simulink model "ROSCO"  (R2023a)
settings: Solver=ode4  StartTime=0.0  StopTime=TMax  FixedStep=simu.dt  RelTol=1e-3  EnableMultiTasking=on
undefined symbols (not defined in the file): DiscIntNeverNeededParam, F, OutList, Parameter, R, rpm2radps, simu, strmatch
libraries: simulink x10
(part 2 of 3)

== system ROSCO/Cyclic Pitch controller/1P Cyclic Pitch Controller1/1P IPCDQ Filtering1/Moving 3P Notch Man Z ==
  Input : Inport
  GenSpeedIN : Inport  Port=2
  Gain : Gain  Gain=1/Parameter.Turbine.G * rpm2radps(1) * 3
  Moving 3P Filt Manual : Subsystem
  Slow Low Pass for Param : DiscreteStateSpace  A=Parameter.Control.cIPC.dLPF_slow.a  B=Parameter.Control.cIPC.dLPF_slow.b  C=Parameter.Control.cIPC.dLPF_slow.c  D=Parameter.Control.cIPC.dLPF_slow.d  SampleTime=Parameter.Control.DT
  Output : Outport  VectorParamsAs1DForOutWhenUnconnected=off
  wires:
  Moving 3P Filt Manual/1(Out1) -> Output/1
  GenSpeedIN/1 -> Slow Low Pass for Param/1
  Input/1 -> Moving 3P Filt Manual/1(u)
  Gain/1 -> Moving 3P Filt Manual/2(rot speed (rad/s))
  Slow Low Pass for Param/1 -> Gain/1

== system ROSCO/Cyclic Pitch controller/1P Cyclic Pitch Controller1/1P IPCDQ Filtering1/Moving 6P Notch Man Y ==
  Input : Inport
  GenSpeedIN : Inport  Port=2
  Gain : Gain  Gain=1/Parameter.Turbine.G * rpm2radps(1) * 3
  Moving 6P Filt Manual : Subsystem
  Slow Low Pass for Param : DiscreteStateSpace  A=Parameter.Control.cIPC.dLPF_slow.a  B=Parameter.Control.cIPC.dLPF_slow.b  C=Parameter.Control.cIPC.dLPF_slow.c  D=Parameter.Control.cIPC.dLPF_slow.d  SampleTime=Parameter.Control.DT
  Output : Outport  VectorParamsAs1DForOutWhenUnconnected=off
  wires:
  Moving 6P Filt Manual/1(Out1) -> Output/1
  GenSpeedIN/1 -> Slow Low Pass for Param/1
  Input/1 -> Moving 6P Filt Manual/1(u)
  Gain/1 -> Moving 6P Filt Manual/2(rot speed (rad/s))
  Slow Low Pass for Param/1 -> Gain/1

== system ROSCO/Cyclic Pitch controller/1P Cyclic Pitch Controller1/1P IPCDQ Filtering1/Moving 6P Notch Man Z ==
  Input : Inport
  GenSpeedIN : Inport  Port=2
  Gain : Gain  Gain=1/Parameter.Turbine.G * rpm2radps(1) * 3
  Moving 6P Filt Manual : Subsystem
  Slow Low Pass for Param : DiscreteStateSpace  A=Parameter.Control.cIPC.dLPF_slow.a  B=Parameter.Control.cIPC.dLPF_slow.b  C=Parameter.Control.cIPC.dLPF_slow.c  D=Parameter.Control.cIPC.dLPF_slow.d  SampleTime=Parameter.Control.DT
  Output : Outport  VectorParamsAs1DForOutWhenUnconnected=off
  wires:
  Slow Low Pass for Param/1 -> Gain/1
  Gain/1 -> Moving 6P Filt Manual/2(rot speed (rad/s))
  Input/1 -> Moving 6P Filt Manual/1(u)
  GenSpeedIN/1 -> Slow Low Pass for Param/1
  Moving 6P Filt Manual/1(Out1) -> Output/1

== system ROSCO/Cyclic Pitch controller/1P Cyclic Pitch Controller1/M0 Signal Proc.1/Moving 1P Notch Man ==
  Input : Inport
  GenSpeedIN : Inport  Port=2
  Gain : Gain  Gain=1/Parameter.Turbine.G * rpm2radps(1)
  Moving 1P Filt Manual : Subsystem
  Slow Low Pass for Param : DiscreteStateSpace  A=Parameter.Control.cIPC.dLPF_slow.a  B=Parameter.Control.cIPC.dLPF_slow.b  C=Parameter.Control.cIPC.dLPF_slow.c  D=Parameter.Control.cIPC.dLPF_slow.d  SampleTime=Parameter.Control.DT
  Output : Outport  VectorParamsAs1DForOutWhenUnconnected=off
  wires:
  GenSpeedIN/1 -> Slow Low Pass for Param/1
  Input/1 -> Moving 1P Filt Manual/1(u)
  Gain/1 -> Moving 1P Filt Manual/2(rot speed (rad/s))
  Slow Low Pass for Param/1 -> Gain/1
  Moving 1P Filt Manual/1(Out1) -> Output/1

== system ROSCO/Cyclic Pitch controller/1P Cyclic Pitch Controller1/M0 Signal Proc.1/Moving 3P Notch Man ==
  Input : Inport
  GenSpeedIN : Inport  Port=2
  Gain : Gain  Gain=1/Parameter.Turbine.G * rpm2radps(1) * 3
  Moving 3P Filt Manual : Subsystem
  Slow Low Pass for Param : DiscreteStateSpace  A=Parameter.Control.cIPC.dLPF_slow.a  B=Parameter.Control.cIPC.dLPF_slow.b  C=Parameter.Control.cIPC.dLPF_slow.c  D=Parameter.Control.cIPC.dLPF_slow.d  SampleTime=Parameter.Control.DT
  Output : Outport  VectorParamsAs1DForOutWhenUnconnected=off
  wires:
  Slow Low Pass for Param/1 -> Gain/1
  Gain/1 -> Moving 3P Filt Manual/2(rot speed (rad/s))
  Input/1 -> Moving 3P Filt Manual/1(u)
  GenSpeedIN/1 -> Slow Low Pass for Param/1
  Moving 3P Filt Manual/1(Out1) -> Output/1

== system ROSCO/Cyclic Pitch controller/2P Cyclic Pitch Controller2/1P IPCDQ Filtering1/Moving 3P Notch Man Y ==
  Input : Inport
  GenSpeedIN : Inport  Port=2
  Gain : Gain  Gain=1/Parameter.Turbine.G * rpm2radps(1) * 3
  Moving 3P Filt Manual : Subsystem
  Slow Low Pass for Param : DiscreteStateSpace  A=Parameter.Control.cIPC.dLPF_slow.a  B=Parameter.Control.cIPC.dLPF_slow.b  C=Parameter.Control.cIPC.dLPF_slow.c  D=Parameter.Control.cIPC.dLPF_slow.d  SampleTime=Parameter.Control.DT
  Output : Outport  VectorParamsAs1DForOutWhenUnconnected=off
  wires:
  Slow Low Pass for Param/1 -> Gain/1
  Gain/1 -> Moving 3P Filt Manual/2(rot speed (rad/s))
  Input/1 -> Moving 3P Filt Manual/1(u)
  GenSpeedIN/1 -> Slow Low Pass for Param/1
  Moving 3P Filt Manual/1(Out1) -> Output/1

== system ROSCO/Cyclic Pitch controller/2P Cyclic Pitch Controller2/1P IPCDQ Filtering1/Moving 3P Notch Man Z ==
  Input : Inport
  GenSpeedIN : Inport  Port=2
  Gain : Gain  Gain=1/Parameter.Turbine.G * rpm2radps(1) * 3
  Moving 3P Filt Manual : Subsystem
  Slow Low Pass for Param : DiscreteStateSpace  A=Parameter.Control.cIPC.dLPF_slow.a  B=Parameter.Control.cIPC.dLPF_slow.b  C=Parameter.Control.cIPC.dLPF_slow.c  D=Parameter.Control.cIPC.dLPF_slow.d  SampleTime=Parameter.Control.DT
  Output : Outport  VectorParamsAs1DForOutWhenUnconnected=off
  wires:
  Moving 3P Filt Manual/1(Out1) -> Output/1
  GenSpeedIN/1 -> Slow Low Pass for Param/1
  Input/1 -> Moving 3P Filt Manual/1(u)
  Gain/1 -> Moving 3P Filt Manual/2(rot speed (rad/s))
  Slow Low Pass for Param/1 -> Gain/1

== system ROSCO/Cyclic Pitch controller/2P Cyclic Pitch Controller2/1P IPCDQ Filtering1/Moving 6P Notch Man Y ==
  Input : Inport
  GenSpeedIN : Inport  Port=2
  Gain : Gain  Gain=1/Parameter.Turbine.G * rpm2radps(1) * 3
  Moving 6P Filt Manual : Subsystem
  Slow Low Pass for Param : DiscreteStateSpace  A=Parameter.Control.cIPC.dLPF_slow.a  B=Parameter.Control.cIPC.dLPF_slow.b  C=Parameter.Control.cIPC.dLPF_slow.c  D=Parameter.Control.cIPC.dLPF_slow.d  SampleTime=Parameter.Control.DT
  Output : Outport  VectorParamsAs1DForOutWhenUnconnected=off
  wires:
  Moving 6P Filt Manual/1(Out1) -> Output/1
  GenSpeedIN/1 -> Slow Low Pass for Param/1
  Input/1 -> Moving 6P Filt Manual/1(u)
  Gain/1 -> Moving 6P Filt Manual/2(rot speed (rad/s))
  Slow Low Pass for Param/1 -> Gain/1

== system ROSCO/Cyclic Pitch controller/2P Cyclic Pitch Controller2/1P IPCDQ Filtering1/Moving 6P Notch Man Z ==
  Input : Inport
  GenSpeedIN : Inport  Port=2
  Gain : Gain  Gain=1/Parameter.Turbine.G * rpm2radps(1) * 3
  Moving 6P Filt Manual : Subsystem
  Slow Low Pass for Param : DiscreteStateSpace  A=Parameter.Control.cIPC.dLPF_slow.a  B=Parameter.Control.cIPC.dLPF_slow.b  C=Parameter.Control.cIPC.dLPF_slow.c  D=Parameter.Control.cIPC.dLPF_slow.d  SampleTime=Parameter.Control.DT
  Output : Outport  VectorParamsAs1DForOutWhenUnconnected=off
  wires:
  Slow Low Pass for Param/1 -> Gain/1
  Gain/1 -> Moving 6P Filt Manual/2(rot speed (rad/s))
  Input/1 -> Moving 6P Filt Manual/1(u)
  GenSpeedIN/1 -> Slow Low Pass for Param/1
  Moving 6P Filt Manual/1(Out1) -> Output/1

== system ROSCO/Cyclic Pitch controller/2P Cyclic Pitch Controller2/M0 Signal Proc.1/Moving 1P Notch Man ==
  Input : Inport
  GenSpeedIN : Inport  Port=2
  Gain : Gain  Gain=1/Parameter.Turbine.G * rpm2radps(1)
  Moving 1P Filt Manual : Subsystem
  Slow Low Pass for Param : DiscreteStateSpace  A=Parameter.Control.cIPC.dLPF_slow.a  B=Parameter.Control.cIPC.dLPF_slow.b  C=Parameter.Control.cIPC.dLPF_slow.c  D=Parameter.Control.cIPC.dLPF_slow.d  SampleTime=Parameter.Control.DT
  Output : Outport  VectorParamsAs1DForOutWhenUnconnected=off
  wires:
  GenSpeedIN/1 -> Slow Low Pass for Param/1
  Input/1 -> Moving 1P Filt Manual/1(u)
  Gain/1 -> Moving 1P Filt Manual/2(rot speed (rad/s))
  Slow Low Pass for Param/1 -> Gain/1
  Moving 1P Filt Manual/1(Out1) -> Output/1

== system ROSCO/Cyclic Pitch controller/2P Cyclic Pitch Controller2/M0 Signal Proc.1/Moving 3P Notch Man ==
  Input : Inport
  GenSpeedIN : Inport  Port=2
  Gain : Gain  Gain=1/Parameter.Turbine.G * rpm2radps(1) * 3
  Moving 3P Filt Manual : Subsystem
  Slow Low Pass for Param : DiscreteStateSpace  A=Parameter.Control.cIPC.dLPF_slow.a  B=Parameter.Control.cIPC.dLPF_slow.b  C=Parameter.Control.cIPC.dLPF_slow.c  D=Parameter.Control.cIPC.dLPF_slow.d  SampleTime=Parameter.Control.DT
  Output : Outport  VectorParamsAs1DForOutWhenUnconnected=off
  wires:
  Slow Low Pass for Param/1 -> Gain/1
  Gain/1 -> Moving 3P Filt Manual/2(rot speed (rad/s))
  Input/1 -> Moving 3P Filt Manual/1(u)
  GenSpeedIN/1 -> Slow Low Pass for Param/1
  Moving 3P Filt Manual/1(Out1) -> Output/1

== system ROSCO/Cyclic Pitch controller/1P Cyclic Pitch Controller1/1P IPCDQ Filtering1/Moving 3P Notch Man Y/Moving 3P Filt Manual ==
  u : Inport
  rot speed (rad/s) : Inport  Port=2
  Den LPV : Subsystem
  Discrete Filter : DiscreteFilter  NumeratorSource=Input port  DenominatorSource=Input port  a0EqualsOne=on
      settings: InputPortMap=u0,p1,p3
  Num LPV : Subsystem
  Out1 : Outport  VectorParamsAs1DForOutWhenUnconnected=off
  wires:
  u/1 -> Discrete Filter/1
  Num LPV/1(b) -> Discrete Filter/2
  Discrete Filter/1 -> Out1/1
  rot speed (rad/s)/1 -> Den LPV/1(rot speed (rad/s)), Num LPV/1(rot speed (rad/s))
  Den LPV/1(a) -> Discrete Filter/3

== system ROSCO/Cyclic Pitch controller/1P Cyclic Pitch Controller1/1P IPCDQ Filtering1/Moving 3P Notch Man Z/Moving 3P Filt Manual ==
  u : Inport
  rot speed (rad/s) : Inport  Port=2
  Den LPV : Subsystem
  Discrete Filter : DiscreteFilter  NumeratorSource=Input port  DenominatorSource=Input port  a0EqualsOne=on
      settings: InputPortMap=u0,p1,p3
  Num LPV : Subsystem
  Out1 : Outport  VectorParamsAs1DForOutWhenUnconnected=off
  wires:
  Den LPV/1(a) -> Discrete Filter/3
  rot speed (rad/s)/1 -> Num LPV/1(rot speed (rad/s)), Den LPV/1(rot speed (rad/s))
  Discrete Filter/1 -> Out1/1
  Num LPV/1(b) -> Discrete Filter/2
  u/1 -> Discrete Filter/1

== system ROSCO/Cyclic Pitch controller/1P Cyclic Pitch Controller1/1P IPCDQ Filtering1/Moving 6P Notch Man Y/Moving 6P Filt Manual ==
  u : Inport
  rot speed (rad/s) : Inport  Port=2
  Den LPV : Subsystem
  Discrete Filter : DiscreteFilter  NumeratorSource=Input port  DenominatorSource=Input port  a0EqualsOne=on
      settings: InputPortMap=u0,p1,p3
  Num LPV : Subsystem
  Out1 : Outport  VectorParamsAs1DForOutWhenUnconnected=off
  wires:
  Den LPV/1(a) -> Discrete Filter/3
  rot speed (rad/s)/1 -> Num LPV/1(rot speed (rad/s)), Den LPV/1(rot speed (rad/s))
  Discrete Filter/1 -> Out1/1
  Num LPV/1(b) -> Discrete Filter/2
  u/1 -> Discrete Filter/1

== system ROSCO/Cyclic Pitch controller/1P Cyclic Pitch Controller1/1P IPCDQ Filtering1/Moving 6P Notch Man Z/Moving 6P Filt Manual ==
  u : Inport
  rot speed (rad/s) : Inport  Port=2
  Den LPV : Subsystem
  Discrete Filter : DiscreteFilter  NumeratorSource=Input port  DenominatorSource=Input port  a0EqualsOne=on
      settings: InputPortMap=u0,p1,p3
  Num LPV : Subsystem
  Out1 : Outport  VectorParamsAs1DForOutWhenUnconnected=off
  wires:
  u/1 -> Discrete Filter/1
  Num LPV/1(b) -> Discrete Filter/2
  Discrete Filter/1 -> Out1/1
  rot speed (rad/s)/1 -> Den LPV/1(rot speed (rad/s)), Num LPV/1(rot speed (rad/s))
  Den LPV/1(a) -> Discrete Filter/3

== system ROSCO/Cyclic Pitch controller/1P Cyclic Pitch Controller1/M0 Signal Proc.1/Moving 1P Notch Man/Moving 1P Filt Manual ==
  u : Inport
  rot speed (rad/s) : Inport  Port=2
  Den LPV : Subsystem
  Discrete Filter : DiscreteFilter  NumeratorSource=Input port  DenominatorSource=Input port  a0EqualsOne=on
      settings: InputPortMap=u0,p1,p3
  Num LPV : Subsystem
  Out1 : Outport  VectorParamsAs1DForOutWhenUnconnected=off
  wires:
  Den LPV/1(a) -> Discrete Filter/3
  rot speed (rad/s)/1 -> Num LPV/1(rot speed (rad/s)), Den LPV/1(rot speed (rad/s))
  Discrete Filter/1 -> Out1/1
  Num LPV/1(b) -> Discrete Filter/2
  u/1 -> Discrete Filter/1

== system ROSCO/Cyclic Pitch controller/1P Cyclic Pitch Controller1/M0 Signal Proc.1/Moving 3P Notch Man/Moving 3P Filt Manual ==
  u : Inport
  rot speed (rad/s) : Inport  Port=2
  Den LPV : Subsystem
  Discrete Filter : DiscreteFilter  NumeratorSource=Input port  DenominatorSource=Input port  a0EqualsOne=on
      settings: InputPortMap=u0,p1,p3
  Num LPV : Subsystem
  Out1 : Outport  VectorParamsAs1DForOutWhenUnconnected=off
  wires:
  u/1 -> Discrete Filter/1
  Num LPV/1(b) -> Discrete Filter/2
  Discrete Filter/1 -> Out1/1
  rot speed (rad/s)/1 -> Den LPV/1(rot speed (rad/s)), Num LPV/1(rot speed (rad/s))
  Den LPV/1(a) -> Discrete Filter/3

== system ROSCO/Cyclic Pitch controller/2P Cyclic Pitch Controller2/1P IPCDQ Filtering1/Moving 3P Notch Man Y/Moving 3P Filt Manual ==
  u : Inport
  rot speed (rad/s) : Inport  Port=2
  Den LPV : Subsystem
  Discrete Filter : DiscreteFilter  NumeratorSource=Input port  DenominatorSource=Input port  a0EqualsOne=on
      settings: InputPortMap=u0,p1,p3
  Num LPV : Subsystem
  Out1 : Outport  VectorParamsAs1DForOutWhenUnconnected=off
  wires:
  u/1 -> Discrete Filter/1
  Num LPV/1(b) -> Discrete Filter/2
  Discrete Filter/1 -> Out1/1
  rot speed (rad/s)/1 -> Den LPV/1(rot speed (rad/s)), Num LPV/1(rot speed (rad/s))
  Den LPV/1(a) -> Discrete Filter/3

== system ROSCO/Cyclic Pitch controller/2P Cyclic Pitch Controller2/1P IPCDQ Filtering1/Moving 3P Notch Man Z/Moving 3P Filt Manual ==
  u : Inport
  rot speed (rad/s) : Inport  Port=2
  Den LPV : Subsystem
  Discrete Filter : DiscreteFilter  NumeratorSource=Input port  DenominatorSource=Input port  a0EqualsOne=on
      settings: InputPortMap=u0,p1,p3
  Num LPV : Subsystem
  Out1 : Outport  VectorParamsAs1DForOutWhenUnconnected=off
  wires:
  Den LPV/1(a) -> Discrete Filter/3
  rot speed (rad/s)/1 -> Num LPV/1(rot speed (rad/s)), Den LPV/1(rot speed (rad/s))
  Discrete Filter/1 -> Out1/1
  Num LPV/1(b) -> Discrete Filter/2
  u/1 -> Discrete Filter/1

== system ROSCO/Cyclic Pitch controller/2P Cyclic Pitch Controller2/1P IPCDQ Filtering1/Moving 6P Notch Man Y/Moving 6P Filt Manual ==
  u : Inport
  rot speed (rad/s) : Inport  Port=2
  Den LPV : Subsystem
  Discrete Filter : DiscreteFilter  NumeratorSource=Input port  DenominatorSource=Input port  a0EqualsOne=on
      settings: InputPortMap=u0,p1,p3
  Num LPV : Subsystem
  Out1 : Outport  VectorParamsAs1DForOutWhenUnconnected=off
  wires:
  Den LPV/1(a) -> Discrete Filter/3
  rot speed (rad/s)/1 -> Num LPV/1(rot speed (rad/s)), Den LPV/1(rot speed (rad/s))
  Discrete Filter/1 -> Out1/1
  Num LPV/1(b) -> Discrete Filter/2
  u/1 -> Discrete Filter/1

== system ROSCO/Cyclic Pitch controller/2P Cyclic Pitch Controller2/1P IPCDQ Filtering1/Moving 6P Notch Man Z/Moving 6P Filt Manual ==
  u : Inport
  rot speed (rad/s) : Inport  Port=2
  Den LPV : Subsystem
  Discrete Filter : DiscreteFilter  NumeratorSource=Input port  DenominatorSource=Input port  a0EqualsOne=on
      settings: InputPortMap=u0,p1,p3
  Num LPV : Subsystem
  Out1 : Outport  VectorParamsAs1DForOutWhenUnconnected=off
  wires:
  u/1 -> Discrete Filter/1
  Num LPV/1(b) -> Discrete Filter/2
  Discrete Filter/1 -> Out1/1
  rot speed (rad/s)/1 -> Den LPV/1(rot speed (rad/s)), Num LPV/1(rot speed (rad/s))
  Den LPV/1(a) -> Discrete Filter/3

== system ROSCO/Cyclic Pitch controller/2P Cyclic Pitch Controller2/M0 Signal Proc.1/Moving 1P Notch Man/Moving 1P Filt Manual ==
  u : Inport
  rot speed (rad/s) : Inport  Port=2
  Den LPV : Subsystem
  Discrete Filter : DiscreteFilter  NumeratorSource=Input port  DenominatorSource=Input port  a0EqualsOne=on
      settings: InputPortMap=u0,p1,p3
  Num LPV : Subsystem
  Out1 : Outport  VectorParamsAs1DForOutWhenUnconnected=off
  wires:
  Den LPV/1(a) -> Discrete Filter/3
  rot speed (rad/s)/1 -> Num LPV/1(rot speed (rad/s)), Den LPV/1(rot speed (rad/s))
  Discrete Filter/1 -> Out1/1
  Num LPV/1(b) -> Discrete Filter/2
  u/1 -> Discrete Filter/1

== system ROSCO/Cyclic Pitch controller/2P Cyclic Pitch Controller2/M0 Signal Proc.1/Moving 3P Notch Man/Moving 3P Filt Manual ==
  u : Inport
  rot speed (rad/s) : Inport  Port=2
  Den LPV : Subsystem
  Discrete Filter : DiscreteFilter  NumeratorSource=Input port  DenominatorSource=Input port  a0EqualsOne=on
      settings: InputPortMap=u0,p1,p3
  Num LPV : Subsystem
  Out1 : Outport  VectorParamsAs1DForOutWhenUnconnected=off
  wires:
  u/1 -> Discrete Filter/1
  Num LPV/1(b) -> Discrete Filter/2
  Discrete Filter/1 -> Out1/1
  rot speed (rad/s)/1 -> Den LPV/1(rot speed (rad/s)), Num LPV/1(rot speed (rad/s))
  Den LPV/1(a) -> Discrete Filter/3

== system ROSCO/Cyclic Pitch controller/1P Cyclic Pitch Controller1/1P IPCDQ Filtering1/Moving 3P Notch Man Y/Moving 3P Filt Manual/Den LPV ==
  rot speed (rad/s) : Inport
  1-D Lookup Table : Lookup_n-D  NumberOfTableDimensions=1  BreakpointsForDimension1=Parameter.Control.cIPC.PSM0_NF_3P.om_3P  BeginIndexSearchUsingPreviousIndexResult=on  Table=Parameter.Control.cIPC.PSM0_NF_3P.a_2  ExtrapMethod=Clip  InternalRulePriority=Speed  RndMeth=Simplest
  1-D Lookup Table1 : Lookup_n-D  NumberOfTableDimensions=1  BreakpointsForDimension1=Parameter.Control.cIPC.PSM0_NF_3P.om_3P  BeginIndexSearchUsingPreviousIndexResult=on  Table=Parameter.Control.cIPC.PSM0_NF_3P.a_1  ExtrapMethod=Clip  InternalRulePriority=Speed  RndMeth=Simplest
  1-D Lookup Table2 : Lookup_n-D  NumberOfTableDimensions=1  BreakpointsForDimension1=Parameter.Control.cIPC.PSM0_NF_3P.om_3P  BeginIndexSearchUsingPreviousIndexResult=on  Table=Parameter.Control.cIPC.PSM0_NF_3P.a_0  ExtrapMethod=Clip  InternalRulePriority=Speed  RndMeth=Simplest
  Mux : Mux  Inputs=3
  a : Outport  VectorParamsAs1DForOutWhenUnconnected=off
  wires:
  1-D Lookup Table/1 -> Mux/1
  1-D Lookup Table1/1 -> Mux/2
  Mux/1 -> a/1
  rot speed (rad/s)/1 -> 1-D Lookup Table2/1, 1-D Lookup Table/1, 1-D Lookup Table1/1
  1-D Lookup Table2/1 -> Mux/3

== system ROSCO/Cyclic Pitch controller/1P Cyclic Pitch Controller1/1P IPCDQ Filtering1/Moving 3P Notch Man Y/Moving 3P Filt Manual/Num LPV ==
  rot speed (rad/s) : Inport
  1-D Lookup Table : Lookup_n-D  NumberOfTableDimensions=1  BreakpointsForDimension1=Parameter.Control.cIPC.PSM0_NF_3P.om_3P  BeginIndexSearchUsingPreviousIndexResult=on  Table=Parameter.Control.cIPC.PSM0_NF_3P.b_2  ExtrapMethod=Clip  InternalRulePriority=Speed  RndMeth=Simplest
  1-D Lookup Table1 : Lookup_n-D  NumberOfTableDimensions=1  BreakpointsForDimension1=Parameter.Control.cIPC.PSM0_NF_3P.om_3P  BeginIndexSearchUsingPreviousIndexResult=on  Table=Parameter.Control.cIPC.PSM0_NF_3P.b_1  ExtrapMethod=Clip  InternalRulePriority=Speed  RndMeth=Simplest
  1-D Lookup Table2 : Lookup_n-D  NumberOfTableDimensions=1  BreakpointsForDimension1=Parameter.Control.cIPC.PSM0_NF_3P.om_3P  BeginIndexSearchUsingPreviousIndexResult=on  Table=Parameter.Control.cIPC.PSM0_NF_3P.b_0  ExtrapMethod=Clip  InternalRulePriority=Speed  RndMeth=Simplest
  Mux : Mux  Inputs=3
  b : Outport  VectorParamsAs1DForOutWhenUnconnected=off
  wires:
  1-D Lookup Table2/1 -> Mux/3
  rot speed (rad/s)/1 -> 1-D Lookup Table1/1, 1-D Lookup Table/1, 1-D Lookup Table2/1
  Mux/1 -> b/1
  1-D Lookup Table1/1 -> Mux/2
  1-D Lookup Table/1 -> Mux/1

== system ROSCO/Cyclic Pitch controller/1P Cyclic Pitch Controller1/1P IPCDQ Filtering1/Moving 3P Notch Man Z/Moving 3P Filt Manual/Den LPV ==
  rot speed (rad/s) : Inport
  1-D Lookup Table : Lookup_n-D  NumberOfTableDimensions=1  BreakpointsForDimension1=Parameter.Control.cIPC.PSM0_NF_3P.om_3P  BeginIndexSearchUsingPreviousIndexResult=on  Table=Parameter.Control.cIPC.PSM0_NF_3P.a_2  ExtrapMethod=Clip  InternalRulePriority=Speed  RndMeth=Simplest
  1-D Lookup Table1 : Lookup_n-D  NumberOfTableDimensions=1  BreakpointsForDimension1=Parameter.Control.cIPC.PSM0_NF_3P.om_3P  BeginIndexSearchUsingPreviousIndexResult=on  Table=Parameter.Control.cIPC.PSM0_NF_3P.a_1  ExtrapMethod=Clip  InternalRulePriority=Speed  RndMeth=Simplest
  1-D Lookup Table2 : Lookup_n-D  NumberOfTableDimensions=1  BreakpointsForDimension1=Parameter.Control.cIPC.PSM0_NF_3P.om_3P  BeginIndexSearchUsingPreviousIndexResult=on  Table=Parameter.Control.cIPC.PSM0_NF_3P.a_0  ExtrapMethod=Clip  InternalRulePriority=Speed  RndMeth=Simplest
  Mux : Mux  Inputs=3
  a : Outport  VectorParamsAs1DForOutWhenUnconnected=off
  wires:
  1-D Lookup Table2/1 -> Mux/3
  rot speed (rad/s)/1 -> 1-D Lookup Table1/1, 1-D Lookup Table/1, 1-D Lookup Table2/1
  Mux/1 -> a/1
  1-D Lookup Table1/1 -> Mux/2
  1-D Lookup Table/1 -> Mux/1

== system ROSCO/Cyclic Pitch controller/1P Cyclic Pitch Controller1/1P IPCDQ Filtering1/Moving 3P Notch Man Z/Moving 3P Filt Manual/Num LPV ==
  rot speed (rad/s) : Inport
  1-D Lookup Table : Lookup_n-D  NumberOfTableDimensions=1  BreakpointsForDimension1=Parameter.Control.cIPC.PSM0_NF_3P.om_3P  BeginIndexSearchUsingPreviousIndexResult=on  Table=Parameter.Control.cIPC.PSM0_NF_3P.b_2  ExtrapMethod=Clip  InternalRulePriority=Speed  RndMeth=Simplest
  1-D Lookup Table1 : Lookup_n-D  NumberOfTableDimensions=1  BreakpointsForDimension1=Parameter.Control.cIPC.PSM0_NF_3P.om_3P  BeginIndexSearchUsingPreviousIndexResult=on  Table=Parameter.Control.cIPC.PSM0_NF_3P.b_1  ExtrapMethod=Clip  InternalRulePriority=Speed  RndMeth=Simplest
  1-D Lookup Table2 : Lookup_n-D  NumberOfTableDimensions=1  BreakpointsForDimension1=Parameter.Control.cIPC.PSM0_NF_3P.om_3P  BeginIndexSearchUsingPreviousIndexResult=on  Table=Parameter.Control.cIPC.PSM0_NF_3P.b_0  ExtrapMethod=Clip  InternalRulePriority=Speed  RndMeth=Simplest
  Mux : Mux  Inputs=3
  b : Outport  VectorParamsAs1DForOutWhenUnconnected=off
  wires:
  1-D Lookup Table/1 -> Mux/1
  1-D Lookup Table1/1 -> Mux/2
  Mux/1 -> b/1
  rot speed (rad/s)/1 -> 1-D Lookup Table2/1, 1-D Lookup Table/1, 1-D Lookup Table1/1
  1-D Lookup Table2/1 -> Mux/3

== system ROSCO/Cyclic Pitch controller/1P Cyclic Pitch Controller1/1P IPCDQ Filtering1/Moving 6P Notch Man Y/Moving 6P Filt Manual/Den LPV ==
  rot speed (rad/s) : Inport
  1-D Lookup Table : Lookup_n-D  NumberOfTableDimensions=1  BreakpointsForDimension1=Parameter.Control.cIPC.PSM0_NF_6P.om_6P  BeginIndexSearchUsingPreviousIndexResult=on  Table=Parameter.Control.cIPC.PSM0_NF_6P.a_2  ExtrapMethod=Clip  InternalRulePriority=Speed  RndMeth=Simplest
  1-D Lookup Table1 : Lookup_n-D  NumberOfTableDimensions=1  BreakpointsForDimension1=Parameter.Control.cIPC.PSM0_NF_6P.om_6P  BeginIndexSearchUsingPreviousIndexResult=on  Table=Parameter.Control.cIPC.PSM0_NF_6P.a_1  ExtrapMethod=Clip  InternalRulePriority=Speed  RndMeth=Simplest
  1-D Lookup Table2 : Lookup_n-D  NumberOfTableDimensions=1  BreakpointsForDimension1=Parameter.Control.cIPC.PSM0_NF_6P.om_6P  BeginIndexSearchUsingPreviousIndexResult=on  Table=Parameter.Control.cIPC.PSM0_NF_6P.a_0  ExtrapMethod=Clip  InternalRulePriority=Speed  RndMeth=Simplest
  Mux : Mux  Inputs=3
  a : Outport  VectorParamsAs1DForOutWhenUnconnected=off
  wires:
  1-D Lookup Table2/1 -> Mux/3
  rot speed (rad/s)/1 -> 1-D Lookup Table1/1, 1-D Lookup Table/1, 1-D Lookup Table2/1
  Mux/1 -> a/1
  1-D Lookup Table1/1 -> Mux/2
  1-D Lookup Table/1 -> Mux/1

== system ROSCO/Cyclic Pitch controller/1P Cyclic Pitch Controller1/1P IPCDQ Filtering1/Moving 6P Notch Man Y/Moving 6P Filt Manual/Num LPV ==
  rot speed (rad/s) : Inport
  1-D Lookup Table : Lookup_n-D  NumberOfTableDimensions=1  BreakpointsForDimension1=Parameter.Control.cIPC.PSM0_NF_6P.om_6P  BeginIndexSearchUsingPreviousIndexResult=on  Table=Parameter.Control.cIPC.PSM0_NF_6P.b_2  ExtrapMethod=Clip  InternalRulePriority=Speed  RndMeth=Simplest
  1-D Lookup Table1 : Lookup_n-D  NumberOfTableDimensions=1  BreakpointsForDimension1=Parameter.Control.cIPC.PSM0_NF_6P.om_6P  BeginIndexSearchUsingPreviousIndexResult=on  Table=Parameter.Control.cIPC.PSM0_NF_6P.b_1  ExtrapMethod=Clip  InternalRulePriority=Speed  RndMeth=Simplest
  1-D Lookup Table2 : Lookup_n-D  NumberOfTableDimensions=1  BreakpointsForDimension1=Parameter.Control.cIPC.PSM0_NF_6P.om_6P  BeginIndexSearchUsingPreviousIndexResult=on  Table=Parameter.Control.cIPC.PSM0_NF_6P.b_0  ExtrapMethod=Clip  InternalRulePriority=Speed  RndMeth=Simplest
  Mux : Mux  Inputs=3
  b : Outport  VectorParamsAs1DForOutWhenUnconnected=off
  wires:
  1-D Lookup Table/1 -> Mux/1
  1-D Lookup Table1/1 -> Mux/2
  Mux/1 -> b/1
  rot speed (rad/s)/1 -> 1-D Lookup Table2/1, 1-D Lookup Table1/1, 1-D Lookup Table/1
  1-D Lookup Table2/1 -> Mux/3

== system ROSCO/Cyclic Pitch controller/1P Cyclic Pitch Controller1/1P IPCDQ Filtering1/Moving 6P Notch Man Z/Moving 6P Filt Manual/Den LPV ==
  rot speed (rad/s) : Inport
  1-D Lookup Table : Lookup_n-D  NumberOfTableDimensions=1  BreakpointsForDimension1=Parameter.Control.cIPC.PSM0_NF_6P.om_6P  BeginIndexSearchUsingPreviousIndexResult=on  Table=Parameter.Control.cIPC.PSM0_NF_6P.a_2  ExtrapMethod=Clip  InternalRulePriority=Speed  RndMeth=Simplest
  1-D Lookup Table1 : Lookup_n-D  NumberOfTableDimensions=1  BreakpointsForDimension1=Parameter.Control.cIPC.PSM0_NF_6P.om_6P  BeginIndexSearchUsingPreviousIndexResult=on  Table=Parameter.Control.cIPC.PSM0_NF_6P.a_1  ExtrapMethod=Clip  InternalRulePriority=Speed  RndMeth=Simplest
  1-D Lookup Table2 : Lookup_n-D  NumberOfTableDimensions=1  BreakpointsForDimension1=Parameter.Control.cIPC.PSM0_NF_6P.om_6P  BeginIndexSearchUsingPreviousIndexResult=on  Table=Parameter.Control.cIPC.PSM0_NF_6P.a_0  ExtrapMethod=Clip  InternalRulePriority=Speed  RndMeth=Simplest
  Mux : Mux  Inputs=3
  a : Outport  VectorParamsAs1DForOutWhenUnconnected=off
  wires:
  1-D Lookup Table/1 -> Mux/1
  1-D Lookup Table1/1 -> Mux/2
  Mux/1 -> a/1
  rot speed (rad/s)/1 -> 1-D Lookup Table2/1, 1-D Lookup Table/1, 1-D Lookup Table1/1
  1-D Lookup Table2/1 -> Mux/3

== system ROSCO/Cyclic Pitch controller/1P Cyclic Pitch Controller1/1P IPCDQ Filtering1/Moving 6P Notch Man Z/Moving 6P Filt Manual/Num LPV ==
  rot speed (rad/s) : Inport
  1-D Lookup Table : Lookup_n-D  NumberOfTableDimensions=1  BreakpointsForDimension1=Parameter.Control.cIPC.PSM0_NF_6P.om_6P  BeginIndexSearchUsingPreviousIndexResult=on  Table=Parameter.Control.cIPC.PSM0_NF_6P.b_2  ExtrapMethod=Clip  InternalRulePriority=Speed  RndMeth=Simplest
  1-D Lookup Table1 : Lookup_n-D  NumberOfTableDimensions=1  BreakpointsForDimension1=Parameter.Control.cIPC.PSM0_NF_6P.om_6P  BeginIndexSearchUsingPreviousIndexResult=on  Table=Parameter.Control.cIPC.PSM0_NF_6P.b_1  ExtrapMethod=Clip  InternalRulePriority=Speed  RndMeth=Simplest
  1-D Lookup Table2 : Lookup_n-D  NumberOfTableDimensions=1  BreakpointsForDimension1=Parameter.Control.cIPC.PSM0_NF_6P.om_6P  BeginIndexSearchUsingPreviousIndexResult=on  Table=Parameter.Control.cIPC.PSM0_NF_6P.b_0  ExtrapMethod=Clip  InternalRulePriority=Speed  RndMeth=Simplest
  Mux : Mux  Inputs=3
  b : Outport  VectorParamsAs1DForOutWhenUnconnected=off
  wires:
  1-D Lookup Table2/1 -> Mux/3
  rot speed (rad/s)/1 -> 1-D Lookup Table1/1, 1-D Lookup Table/1, 1-D Lookup Table2/1
  Mux/1 -> b/1
  1-D Lookup Table1/1 -> Mux/2
  1-D Lookup Table/1 -> Mux/1

== system ROSCO/Cyclic Pitch controller/1P Cyclic Pitch Controller1/M0 Signal Proc.1/Moving 1P Notch Man/Moving 1P Filt Manual/Den LPV ==
  rot speed (rad/s) : Inport
  1-D Lookup Table : Lookup_n-D  NumberOfTableDimensions=1  BreakpointsForDimension1=Parameter.Control.cIPC.PSM0_NF_1P.om_1P  BeginIndexSearchUsingPreviousIndexResult=on  Table=Parameter.Control.cIPC.PSM0_NF_1P.a_2  ExtrapMethod=Clip  InternalRulePriority=Speed  RndMeth=Simplest
  1-D Lookup Table1 : Lookup_n-D  NumberOfTableDimensions=1  BreakpointsForDimension1=Parameter.Control.cIPC.PSM0_NF_1P.om_1P  BeginIndexSearchUsingPreviousIndexResult=on  Table=Parameter.Control.cIPC.PSM0_NF_1P.a_1  ExtrapMethod=Clip  InternalRulePriority=Speed  RndMeth=Simplest
  1-D Lookup Table2 : Lookup_n-D  NumberOfTableDimensions=1  BreakpointsForDimension1=Parameter.Control.cIPC.PSM0_NF_1P.om_1P  BeginIndexSearchUsingPreviousIndexResult=on  Table=Parameter.Control.cIPC.PSM0_NF_1P.a_0  ExtrapMethod=Clip  InternalRulePriority=Speed  RndMeth=Simplest
  Mux : Mux  Inputs=3
  a : Outport  VectorParamsAs1DForOutWhenUnconnected=off
  wires:
  1-D Lookup Table2/1 -> Mux/3
  rot speed (rad/s)/1 -> 1-D Lookup Table1/1, 1-D Lookup Table/1, 1-D Lookup Table2/1
  Mux/1 -> a/1
  1-D Lookup Table1/1 -> Mux/2
  1-D Lookup Table/1 -> Mux/1

== system ROSCO/Cyclic Pitch controller/1P Cyclic Pitch Controller1/M0 Signal Proc.1/Moving 1P Notch Man/Moving 1P Filt Manual/Num LPV ==
  rot speed (rad/s) : Inport
  1-D Lookup Table : Lookup_n-D  NumberOfTableDimensions=1  BreakpointsForDimension1=Parameter.Control.cIPC.PSM0_NF_1P.om_1P  BeginIndexSearchUsingPreviousIndexResult=on  Table=Parameter.Control.cIPC.PSM0_NF_1P.b_2  ExtrapMethod=Clip  InternalRulePriority=Speed  RndMeth=Simplest
  1-D Lookup Table1 : Lookup_n-D  NumberOfTableDimensions=1  BreakpointsForDimension1=Parameter.Control.cIPC.PSM0_NF_1P.om_1P  BeginIndexSearchUsingPreviousIndexResult=on  Table=Parameter.Control.cIPC.PSM0_NF_1P.b_1  ExtrapMethod=Clip  InternalRulePriority=Speed  RndMeth=Simplest
  1-D Lookup Table2 : Lookup_n-D  NumberOfTableDimensions=1  BreakpointsForDimension1=Parameter.Control.cIPC.PSM0_NF_1P.om_1P  BeginIndexSearchUsingPreviousIndexResult=on  Table=Parameter.Control.cIPC.PSM0_NF_1P.b_0  ExtrapMethod=Clip  InternalRulePriority=Speed  RndMeth=Simplest
  Mux : Mux  Inputs=3
  b : Outport  VectorParamsAs1DForOutWhenUnconnected=off
  wires:
  1-D Lookup Table/1 -> Mux/1
  1-D Lookup Table1/1 -> Mux/2
  Mux/1 -> b/1
  rot speed (rad/s)/1 -> 1-D Lookup Table2/1, 1-D Lookup Table/1, 1-D Lookup Table1/1
  1-D Lookup Table2/1 -> Mux/3

== system ROSCO/Cyclic Pitch controller/1P Cyclic Pitch Controller1/M0 Signal Proc.1/Moving 3P Notch Man/Moving 3P Filt Manual/Den LPV ==
  rot speed (rad/s) : Inport
  1-D Lookup Table : Lookup_n-D  NumberOfTableDimensions=1  BreakpointsForDimension1=Parameter.Control.cIPC.PSM0_NF_3P.om_3P  BeginIndexSearchUsingPreviousIndexResult=on  Table=Parameter.Control.cIPC.PSM0_NF_3P.a_2  ExtrapMethod=Clip  InternalRulePriority=Speed  RndMeth=Simplest
  1-D Lookup Table1 : Lookup_n-D  NumberOfTableDimensions=1  BreakpointsForDimension1=Parameter.Control.cIPC.PSM0_NF_3P.om_3P  BeginIndexSearchUsingPreviousIndexResult=on  Table=Parameter.Control.cIPC.PSM0_NF_3P.a_1  ExtrapMethod=Clip  InternalRulePriority=Speed  RndMeth=Simplest
  1-D Lookup Table2 : Lookup_n-D  NumberOfTableDimensions=1  BreakpointsForDimension1=Parameter.Control.cIPC.PSM0_NF_3P.om_3P  BeginIndexSearchUsingPreviousIndexResult=on  Table=Parameter.Control.cIPC.PSM0_NF_3P.a_0  ExtrapMethod=Clip  InternalRulePriority=Speed  RndMeth=Simplest
  Mux : Mux  Inputs=3
  a : Outport  VectorParamsAs1DForOutWhenUnconnected=off
  wires:
  1-D Lookup Table/1 -> Mux/1
  1-D Lookup Table1/1 -> Mux/2
  Mux/1 -> a/1
  rot speed (rad/s)/1 -> 1-D Lookup Table2/1, 1-D Lookup Table/1, 1-D Lookup Table1/1
  1-D Lookup Table2/1 -> Mux/3

== system ROSCO/Cyclic Pitch controller/1P Cyclic Pitch Controller1/M0 Signal Proc.1/Moving 3P Notch Man/Moving 3P Filt Manual/Num LPV ==
  rot speed (rad/s) : Inport
  1-D Lookup Table : Lookup_n-D  NumberOfTableDimensions=1  BreakpointsForDimension1=Parameter.Control.cIPC.PSM0_NF_3P.om_3P  BeginIndexSearchUsingPreviousIndexResult=on  Table=Parameter.Control.cIPC.PSM0_NF_3P.b_2  ExtrapMethod=Clip  InternalRulePriority=Speed  RndMeth=Simplest
  1-D Lookup Table1 : Lookup_n-D  NumberOfTableDimensions=1  BreakpointsForDimension1=Parameter.Control.cIPC.PSM0_NF_3P.om_3P  BeginIndexSearchUsingPreviousIndexResult=on  Table=Parameter.Control.cIPC.PSM0_NF_3P.b_1  ExtrapMethod=Clip  InternalRulePriority=Speed  RndMeth=Simplest
  1-D Lookup Table2 : Lookup_n-D  NumberOfTableDimensions=1  BreakpointsForDimension1=Parameter.Control.cIPC.PSM0_NF_3P.om_3P  BeginIndexSearchUsingPreviousIndexResult=on  Table=Parameter.Control.cIPC.PSM0_NF_3P.b_0  ExtrapMethod=Clip  InternalRulePriority=Speed  RndMeth=Simplest
  Mux : Mux  Inputs=3
  b : Outport  VectorParamsAs1DForOutWhenUnconnected=off
  wires:
  1-D Lookup Table2/1 -> Mux/3
  rot speed (rad/s)/1 -> 1-D Lookup Table1/1, 1-D Lookup Table/1, 1-D Lookup Table2/1
  Mux/1 -> b/1
  1-D Lookup Table1/1 -> Mux/2
  1-D Lookup Table/1 -> Mux/1

== system ROSCO/Cyclic Pitch controller/2P Cyclic Pitch Controller2/1P IPCDQ Filtering1/Moving 3P Notch Man Y/Moving 3P Filt Manual/Den LPV ==
  rot speed (rad/s) : Inport
  1-D Lookup Table : Lookup_n-D  NumberOfTableDimensions=1  BreakpointsForDimension1=Parameter.Control.cIPC.PSM0_NF_3P.om_3P  BeginIndexSearchUsingPreviousIndexResult=on  Table=Parameter.Control.cIPC.PSM0_NF_3P.a_2  ExtrapMethod=Clip  InternalRulePriority=Speed  RndMeth=Simplest
  1-D Lookup Table1 : Lookup_n-D  NumberOfTableDimensions=1  BreakpointsForDimension1=Parameter.Control.cIPC.PSM0_NF_3P.om_3P  BeginIndexSearchUsingPreviousIndexResult=on  Table=Parameter.Control.cIPC.PSM0_NF_3P.a_1  ExtrapMethod=Clip  InternalRulePriority=Speed  RndMeth=Simplest
  1-D Lookup Table2 : Lookup_n-D  NumberOfTableDimensions=1  BreakpointsForDimension1=Parameter.Control.cIPC.PSM0_NF_3P.om_3P  BeginIndexSearchUsingPreviousIndexResult=on  Table=Parameter.Control.cIPC.PSM0_NF_3P.a_0  ExtrapMethod=Clip  InternalRulePriority=Speed  RndMeth=Simplest
  Mux : Mux  Inputs=3
  a : Outport  VectorParamsAs1DForOutWhenUnconnected=off
  wires:
  1-D Lookup Table/1 -> Mux/1
  1-D Lookup Table1/1 -> Mux/2
  Mux/1 -> a/1
  rot speed (rad/s)/1 -> 1-D Lookup Table2/1, 1-D Lookup Table/1, 1-D Lookup Table1/1
  1-D Lookup Table2/1 -> Mux/3

== system ROSCO/Cyclic Pitch controller/2P Cyclic Pitch Controller2/1P IPCDQ Filtering1/Moving 3P Notch Man Y/Moving 3P Filt Manual/Num LPV ==
  rot speed (rad/s) : Inport
  1-D Lookup Table : Lookup_n-D  NumberOfTableDimensions=1  BreakpointsForDimension1=Parameter.Control.cIPC.PSM0_NF_3P.om_3P  BeginIndexSearchUsingPreviousIndexResult=on  Table=Parameter.Control.cIPC.PSM0_NF_3P.b_2  ExtrapMethod=Clip  InternalRulePriority=Speed  RndMeth=Simplest
  1-D Lookup Table1 : Lookup_n-D  NumberOfTableDimensions=1  BreakpointsForDimension1=Parameter.Control.cIPC.PSM0_NF_3P.om_3P  BeginIndexSearchUsingPreviousIndexResult=on  Table=Parameter.Control.cIPC.PSM0_NF_3P.b_1  ExtrapMethod=Clip  InternalRulePriority=Speed  RndMeth=Simplest
  1-D Lookup Table2 : Lookup_n-D  NumberOfTableDimensions=1  BreakpointsForDimension1=Parameter.Control.cIPC.PSM0_NF_3P.om_3P  BeginIndexSearchUsingPreviousIndexResult=on  Table=Parameter.Control.cIPC.PSM0_NF_3P.b_0  ExtrapMethod=Clip  InternalRulePriority=Speed  RndMeth=Simplest
  Mux : Mux  Inputs=3
  b : Outport  VectorParamsAs1DForOutWhenUnconnected=off
  wires:
  1-D Lookup Table2/1 -> Mux/3
  rot speed (rad/s)/1 -> 1-D Lookup Table1/1, 1-D Lookup Table/1, 1-D Lookup Table2/1
  Mux/1 -> b/1
  1-D Lookup Table1/1 -> Mux/2
  1-D Lookup Table/1 -> Mux/1

== system ROSCO/Cyclic Pitch controller/2P Cyclic Pitch Controller2/1P IPCDQ Filtering1/Moving 3P Notch Man Z/Moving 3P Filt Manual/Den LPV ==
  rot speed (rad/s) : Inport
  1-D Lookup Table : Lookup_n-D  NumberOfTableDimensions=1  BreakpointsForDimension1=Parameter.Control.cIPC.PSM0_NF_3P.om_3P  BeginIndexSearchUsingPreviousIndexResult=on  Table=Parameter.Control.cIPC.PSM0_NF_3P.a_2  ExtrapMethod=Clip  InternalRulePriority=Speed  RndMeth=Simplest
  1-D Lookup Table1 : Lookup_n-D  NumberOfTableDimensions=1  BreakpointsForDimension1=Parameter.Control.cIPC.PSM0_NF_3P.om_3P  BeginIndexSearchUsingPreviousIndexResult=on  Table=Parameter.Control.cIPC.PSM0_NF_3P.a_1  ExtrapMethod=Clip  InternalRulePriority=Speed  RndMeth=Simplest
  1-D Lookup Table2 : Lookup_n-D  NumberOfTableDimensions=1  BreakpointsForDimension1=Parameter.Control.cIPC.PSM0_NF_3P.om_3P  BeginIndexSearchUsingPreviousIndexResult=on  Table=Parameter.Control.cIPC.PSM0_NF_3P.a_0  ExtrapMethod=Clip  InternalRulePriority=Speed  RndMeth=Simplest
  Mux : Mux  Inputs=3
  a : Outport  VectorParamsAs1DForOutWhenUnconnected=off
  wires:
  1-D Lookup Table2/1 -> Mux/3
  rot speed (rad/s)/1 -> 1-D Lookup Table1/1, 1-D Lookup Table/1, 1-D Lookup Table2/1
  Mux/1 -> a/1
  1-D Lookup Table1/1 -> Mux/2
  1-D Lookup Table/1 -> Mux/1

== system ROSCO/Cyclic Pitch controller/2P Cyclic Pitch Controller2/1P IPCDQ Filtering1/Moving 3P Notch Man Z/Moving 3P Filt Manual/Num LPV ==
  rot speed (rad/s) : Inport
  1-D Lookup Table : Lookup_n-D  NumberOfTableDimensions=1  BreakpointsForDimension1=Parameter.Control.cIPC.PSM0_NF_3P.om_3P  BeginIndexSearchUsingPreviousIndexResult=on  Table=Parameter.Control.cIPC.PSM0_NF_3P.b_2  ExtrapMethod=Clip  InternalRulePriority=Speed  RndMeth=Simplest
  1-D Lookup Table1 : Lookup_n-D  NumberOfTableDimensions=1  BreakpointsForDimension1=Parameter.Control.cIPC.PSM0_NF_3P.om_3P  BeginIndexSearchUsingPreviousIndexResult=on  Table=Parameter.Control.cIPC.PSM0_NF_3P.b_1  ExtrapMethod=Clip  InternalRulePriority=Speed  RndMeth=Simplest
  1-D Lookup Table2 : Lookup_n-D  NumberOfTableDimensions=1  BreakpointsForDimension1=Parameter.Control.cIPC.PSM0_NF_3P.om_3P  BeginIndexSearchUsingPreviousIndexResult=on  Table=Parameter.Control.cIPC.PSM0_NF_3P.b_0  ExtrapMethod=Clip  InternalRulePriority=Speed  RndMeth=Simplest
  Mux : Mux  Inputs=3
  b : Outport  VectorParamsAs1DForOutWhenUnconnected=off
  wires:
  1-D Lookup Table/1 -> Mux/1
  1-D Lookup Table1/1 -> Mux/2
  Mux/1 -> b/1
  rot speed (rad/s)/1 -> 1-D Lookup Table2/1, 1-D Lookup Table/1, 1-D Lookup Table1/1
  1-D Lookup Table2/1 -> Mux/3

== system ROSCO/Cyclic Pitch controller/2P Cyclic Pitch Controller2/1P IPCDQ Filtering1/Moving 6P Notch Man Y/Moving 6P Filt Manual/Den LPV ==
  rot speed (rad/s) : Inport
  1-D Lookup Table : Lookup_n-D  NumberOfTableDimensions=1  BreakpointsForDimension1=Parameter.Control.cIPC.PSM0_NF_6P.om_6P  BeginIndexSearchUsingPreviousIndexResult=on  Table=Parameter.Control.cIPC.PSM0_NF_6P.a_2  ExtrapMethod=Clip  InternalRulePriority=Speed  RndMeth=Simplest
  1-D Lookup Table1 : Lookup_n-D  NumberOfTableDimensions=1  BreakpointsForDimension1=Parameter.Control.cIPC.PSM0_NF_6P.om_6P  BeginIndexSearchUsingPreviousIndexResult=on  Table=Parameter.Control.cIPC.PSM0_NF_6P.a_1  ExtrapMethod=Clip  InternalRulePriority=Speed  RndMeth=Simplest
  1-D Lookup Table2 : Lookup_n-D  NumberOfTableDimensions=1  BreakpointsForDimension1=Parameter.Control.cIPC.PSM0_NF_6P.om_6P  BeginIndexSearchUsingPreviousIndexResult=on  Table=Parameter.Control.cIPC.PSM0_NF_6P.a_0  ExtrapMethod=Clip  InternalRulePriority=Speed  RndMeth=Simplest
  Mux : Mux  Inputs=3
  a : Outport  VectorParamsAs1DForOutWhenUnconnected=off
  wires:
  1-D Lookup Table2/1 -> Mux/3
  rot speed (rad/s)/1 -> 1-D Lookup Table1/1, 1-D Lookup Table/1, 1-D Lookup Table2/1
  Mux/1 -> a/1
  1-D Lookup Table1/1 -> Mux/2
  1-D Lookup Table/1 -> Mux/1

== system ROSCO/Cyclic Pitch controller/2P Cyclic Pitch Controller2/1P IPCDQ Filtering1/Moving 6P Notch Man Y/Moving 6P Filt Manual/Num LPV ==
  rot speed (rad/s) : Inport
  1-D Lookup Table : Lookup_n-D  NumberOfTableDimensions=1  BreakpointsForDimension1=Parameter.Control.cIPC.PSM0_NF_6P.om_6P  BeginIndexSearchUsingPreviousIndexResult=on  Table=Parameter.Control.cIPC.PSM0_NF_6P.b_2  ExtrapMethod=Clip  InternalRulePriority=Speed  RndMeth=Simplest
  1-D Lookup Table1 : Lookup_n-D  NumberOfTableDimensions=1  BreakpointsForDimension1=Parameter.Control.cIPC.PSM0_NF_6P.om_6P  BeginIndexSearchUsingPreviousIndexResult=on  Table=Parameter.Control.cIPC.PSM0_NF_6P.b_1  ExtrapMethod=Clip  InternalRulePriority=Speed  RndMeth=Simplest
  1-D Lookup Table2 : Lookup_n-D  NumberOfTableDimensions=1  BreakpointsForDimension1=Parameter.Control.cIPC.PSM0_NF_6P.om_6P  BeginIndexSearchUsingPreviousIndexResult=on  Table=Parameter.Control.cIPC.PSM0_NF_6P.b_0  ExtrapMethod=Clip  InternalRulePriority=Speed  RndMeth=Simplest
  Mux : Mux  Inputs=3
  b : Outport  VectorParamsAs1DForOutWhenUnconnected=off
  wires:
  1-D Lookup Table/1 -> Mux/1
  1-D Lookup Table1/1 -> Mux/2
  Mux/1 -> b/1
  rot speed (rad/s)/1 -> 1-D Lookup Table2/1, 1-D Lookup Table1/1, 1-D Lookup Table/1
  1-D Lookup Table2/1 -> Mux/3

== system ROSCO/Cyclic Pitch controller/2P Cyclic Pitch Controller2/1P IPCDQ Filtering1/Moving 6P Notch Man Z/Moving 6P Filt Manual/Den LPV ==
  rot speed (rad/s) : Inport
  1-D Lookup Table : Lookup_n-D  NumberOfTableDimensions=1  BreakpointsForDimension1=Parameter.Control.cIPC.PSM0_NF_6P.om_6P  BeginIndexSearchUsingPreviousIndexResult=on  Table=Parameter.Control.cIPC.PSM0_NF_6P.a_2  ExtrapMethod=Clip  InternalRulePriority=Speed  RndMeth=Simplest
  1-D Lookup Table1 : Lookup_n-D  NumberOfTableDimensions=1  BreakpointsForDimension1=Parameter.Control.cIPC.PSM0_NF_6P.om_6P  BeginIndexSearchUsingPreviousIndexResult=on  Table=Parameter.Control.cIPC.PSM0_NF_6P.a_1  ExtrapMethod=Clip  InternalRulePriority=Speed  RndMeth=Simplest
  1-D Lookup Table2 : Lookup_n-D  NumberOfTableDimensions=1  BreakpointsForDimension1=Parameter.Control.cIPC.PSM0_NF_6P.om_6P  BeginIndexSearchUsingPreviousIndexResult=on  Table=Parameter.Control.cIPC.PSM0_NF_6P.a_0  ExtrapMethod=Clip  InternalRulePriority=Speed  RndMeth=Simplest
  Mux : Mux  Inputs=3
  a : Outport  VectorParamsAs1DForOutWhenUnconnected=off
  wires:
  1-D Lookup Table/1 -> Mux/1
  1-D Lookup Table1/1 -> Mux/2
  Mux/1 -> a/1
  rot speed (rad/s)/1 -> 1-D Lookup Table2/1, 1-D Lookup Table/1, 1-D Lookup Table1/1
  1-D Lookup Table2/1 -> Mux/3

== system ROSCO/Cyclic Pitch controller/2P Cyclic Pitch Controller2/1P IPCDQ Filtering1/Moving 6P Notch Man Z/Moving 6P Filt Manual/Num LPV ==
  rot speed (rad/s) : Inport
  1-D Lookup Table : Lookup_n-D  NumberOfTableDimensions=1  BreakpointsForDimension1=Parameter.Control.cIPC.PSM0_NF_6P.om_6P  BeginIndexSearchUsingPreviousIndexResult=on  Table=Parameter.Control.cIPC.PSM0_NF_6P.b_2  ExtrapMethod=Clip  InternalRulePriority=Speed  RndMeth=Simplest
  1-D Lookup Table1 : Lookup_n-D  NumberOfTableDimensions=1  BreakpointsForDimension1=Parameter.Control.cIPC.PSM0_NF_6P.om_6P  BeginIndexSearchUsingPreviousIndexResult=on  Table=Parameter.Control.cIPC.PSM0_NF_6P.b_1  ExtrapMethod=Clip  InternalRulePriority=Speed  RndMeth=Simplest
  1-D Lookup Table2 : Lookup_n-D  NumberOfTableDimensions=1  BreakpointsForDimension1=Parameter.Control.cIPC.PSM0_NF_6P.om_6P  BeginIndexSearchUsingPreviousIndexResult=on  Table=Parameter.Control.cIPC.PSM0_NF_6P.b_0  ExtrapMethod=Clip  InternalRulePriority=Speed  RndMeth=Simplest
  Mux : Mux  Inputs=3
  b : Outport  VectorParamsAs1DForOutWhenUnconnected=off
  wires:
  1-D Lookup Table2/1 -> Mux/3
  rot speed (rad/s)/1 -> 1-D Lookup Table1/1, 1-D Lookup Table/1, 1-D Lookup Table2/1
  Mux/1 -> b/1
  1-D Lookup Table1/1 -> Mux/2
  1-D Lookup Table/1 -> Mux/1

== system ROSCO/Cyclic Pitch controller/2P Cyclic Pitch Controller2/M0 Signal Proc.1/Moving 1P Notch Man/Moving 1P Filt Manual/Den LPV ==
  rot speed (rad/s) : Inport
  1-D Lookup Table : Lookup_n-D  NumberOfTableDimensions=1  BreakpointsForDimension1=Parameter.Control.cIPC.PSM0_NF_1P.om_1P  BeginIndexSearchUsingPreviousIndexResult=on  Table=Parameter.Control.cIPC.PSM0_NF_1P.a_2  ExtrapMethod=Clip  InternalRulePriority=Speed  RndMeth=Simplest
  1-D Lookup Table1 : Lookup_n-D  NumberOfTableDimensions=1  BreakpointsForDimension1=Parameter.Control.cIPC.PSM0_NF_1P.om_1P  BeginIndexSearchUsingPreviousIndexResult=on  Table=Parameter.Control.cIPC.PSM0_NF_1P.a_1  ExtrapMethod=Clip  InternalRulePriority=Speed  RndMeth=Simplest
  1-D Lookup Table2 : Lookup_n-D  NumberOfTableDimensions=1  BreakpointsForDimension1=Parameter.Control.cIPC.PSM0_NF_1P.om_1P  BeginIndexSearchUsingPreviousIndexResult=on  Table=Parameter.Control.cIPC.PSM0_NF_1P.a_0  ExtrapMethod=Clip  InternalRulePriority=Speed  RndMeth=Simplest
  Mux : Mux  Inputs=3
  a : Outport  VectorParamsAs1DForOutWhenUnconnected=off
  wires:
  1-D Lookup Table2/1 -> Mux/3
  rot speed (rad/s)/1 -> 1-D Lookup Table1/1, 1-D Lookup Table/1, 1-D Lookup Table2/1
  Mux/1 -> a/1
  1-D Lookup Table1/1 -> Mux/2
  1-D Lookup Table/1 -> Mux/1

== system ROSCO/Cyclic Pitch controller/2P Cyclic Pitch Controller2/M0 Signal Proc.1/Moving 1P Notch Man/Moving 1P Filt Manual/Num LPV ==
  rot speed (rad/s) : Inport
  1-D Lookup Table : Lookup_n-D  NumberOfTableDimensions=1  BreakpointsForDimension1=Parameter.Control.cIPC.PSM0_NF_1P.om_1P  BeginIndexSearchUsingPreviousIndexResult=on  Table=Parameter.Control.cIPC.PSM0_NF_1P.b_2  ExtrapMethod=Clip  InternalRulePriority=Speed  RndMeth=Simplest
  1-D Lookup Table1 : Lookup_n-D  NumberOfTableDimensions=1  BreakpointsForDimension1=Parameter.Control.cIPC.PSM0_NF_1P.om_1P  BeginIndexSearchUsingPreviousIndexResult=on  Table=Parameter.Control.cIPC.PSM0_NF_1P.b_1  ExtrapMethod=Clip  InternalRulePriority=Speed  RndMeth=Simplest
  1-D Lookup Table2 : Lookup_n-D  NumberOfTableDimensions=1  BreakpointsForDimension1=Parameter.Control.cIPC.PSM0_NF_1P.om_1P  BeginIndexSearchUsingPreviousIndexResult=on  Table=Parameter.Control.cIPC.PSM0_NF_1P.b_0  ExtrapMethod=Clip  InternalRulePriority=Speed  RndMeth=Simplest
  Mux : Mux  Inputs=3
  b : Outport  VectorParamsAs1DForOutWhenUnconnected=off
  wires:
  1-D Lookup Table/1 -> Mux/1
  1-D Lookup Table1/1 -> Mux/2
  Mux/1 -> b/1
  rot speed (rad/s)/1 -> 1-D Lookup Table2/1, 1-D Lookup Table/1, 1-D Lookup Table1/1
  1-D Lookup Table2/1 -> Mux/3

== system ROSCO/Cyclic Pitch controller/2P Cyclic Pitch Controller2/M0 Signal Proc.1/Moving 3P Notch Man/Moving 3P Filt Manual/Den LPV ==
  rot speed (rad/s) : Inport
  1-D Lookup Table : Lookup_n-D  NumberOfTableDimensions=1  BreakpointsForDimension1=Parameter.Control.cIPC.PSM0_NF_3P.om_3P  BeginIndexSearchUsingPreviousIndexResult=on  Table=Parameter.Control.cIPC.PSM0_NF_3P.a_2  ExtrapMethod=Clip  InternalRulePriority=Speed  RndMeth=Simplest
  1-D Lookup Table1 : Lookup_n-D  NumberOfTableDimensions=1  BreakpointsForDimension1=Parameter.Control.cIPC.PSM0_NF_3P.om_3P  BeginIndexSearchUsingPreviousIndexResult=on  Table=Parameter.Control.cIPC.PSM0_NF_3P.a_1  ExtrapMethod=Clip  InternalRulePriority=Speed  RndMeth=Simplest
  1-D Lookup Table2 : Lookup_n-D  NumberOfTableDimensions=1  BreakpointsForDimension1=Parameter.Control.cIPC.PSM0_NF_3P.om_3P  BeginIndexSearchUsingPreviousIndexResult=on  Table=Parameter.Control.cIPC.PSM0_NF_3P.a_0  ExtrapMethod=Clip  InternalRulePriority=Speed  RndMeth=Simplest
  Mux : Mux  Inputs=3
  a : Outport  VectorParamsAs1DForOutWhenUnconnected=off
  wires:
  1-D Lookup Table/1 -> Mux/1
  1-D Lookup Table1/1 -> Mux/2
  Mux/1 -> a/1
  rot speed (rad/s)/1 -> 1-D Lookup Table2/1, 1-D Lookup Table/1, 1-D Lookup Table1/1
  1-D Lookup Table2/1 -> Mux/3

== system ROSCO/Cyclic Pitch controller/2P Cyclic Pitch Controller2/M0 Signal Proc.1/Moving 3P Notch Man/Moving 3P Filt Manual/Num LPV ==
  rot speed (rad/s) : Inport
  1-D Lookup Table : Lookup_n-D  NumberOfTableDimensions=1  BreakpointsForDimension1=Parameter.Control.cIPC.PSM0_NF_3P.om_3P  BeginIndexSearchUsingPreviousIndexResult=on  Table=Parameter.Control.cIPC.PSM0_NF_3P.b_2  ExtrapMethod=Clip  InternalRulePriority=Speed  RndMeth=Simplest
  1-D Lookup Table1 : Lookup_n-D  NumberOfTableDimensions=1  BreakpointsForDimension1=Parameter.Control.cIPC.PSM0_NF_3P.om_3P  BeginIndexSearchUsingPreviousIndexResult=on  Table=Parameter.Control.cIPC.PSM0_NF_3P.b_1  ExtrapMethod=Clip  InternalRulePriority=Speed  RndMeth=Simplest
  1-D Lookup Table2 : Lookup_n-D  NumberOfTableDimensions=1  BreakpointsForDimension1=Parameter.Control.cIPC.PSM0_NF_3P.om_3P  BeginIndexSearchUsingPreviousIndexResult=on  Table=Parameter.Control.cIPC.PSM0_NF_3P.b_0  ExtrapMethod=Clip  InternalRulePriority=Speed  RndMeth=Simplest
  Mux : Mux  Inputs=3
  b : Outport  VectorParamsAs1DForOutWhenUnconnected=off
  wires:
  1-D Lookup Table2/1 -> Mux/3
  rot speed (rad/s)/1 -> 1-D Lookup Table1/1, 1-D Lookup Table/1, 1-D Lookup Table2/1
  Mux/1 -> b/1
  1-D Lookup Table1/1 -> Mux/2
  1-D Lookup Table/1 -> Mux/1

== matlab function ROSCO/Cyclic Pitch controller/1P Cyclic Pitch Controller1/d-q transformation ==
  data: RootMyb input; M_tilt output; Az input; M_yaw output; NumBl input
function [M_tilt,M_yaw] = fwdMBC2(RootMyb, Az, NumBl)
% This block supports the Embedded MATLAB subset.
% See the help menu for details.

if NumBl == 2
    
    My=RootMyb-mean(RootMyb(1:2)); %remove mean
    
    M_tilt = [cosd(Az) cosd(Az+180) 0]*My;
    M_yaw =  [sind(Az) sind(Az+180) 0]*My;
else
    My=RootMyb-mean(RootMyb); %remove mean
    
    M_tilt = [cosd(Az) cosd(Az+120) cosd(Az+240)]*My;
    M_yaw =  [sind(Az) sind(Az+120) sind(Az+240)]*My;
end

== matlab function ROSCO/Cyclic Pitch controller/1P Cyclic Pitch Controller1/inverse d-q transformation ==
  data: bdq input; b1 output size=1; Az input; b2 output size=1; NumBl input; b3 output size=1
function [b1,b2,b3] = bckMBC2(bdq, Az, NumBl)
% This block supports the Embedded MATLAB subset.
% See the help menu for details.


if NumBl == 2
    
    b1=[cosd(Az) sind(Az)]*bdq;
    b2=[cosd(Az - 180) sind(Az - 180)]*bdq;
    b3=0;
    
else
    b1=[cosd(Az) sind(Az)]*bdq;
    b2=[cosd(Az + 120) sind(Az + 120)]*bdq;
    b3=[cosd(Az + 240) sind(Az + 240)]*bdq;
    
end
